simulink model "ROSsystem"  (R2021a)
settings: Solver=VariableStepAuto  StartTime=0.0  StopTime=10.0  RelTol=1e-3
values from neighbouring files (symbols this model uses):
  Fyf = zeros(1,57)    [FyfLookUpNewCar.m]    (also in Fyf_loopup_table.mat = [-9372.31873381 -9371.87234491 -9368.75632133 -9360.32413915)
  ks = 0    [controller_setup.m]
  SlipAngle = -SlipAngle    [FyfLookUpNewCar.m]    (also in Fyf_loopup_table.mat = [0.153111393254 0.147643129209 0.142174865164 0.13670660112 )
  Ts = 0.1    [controller_setup.m]
  Vx = 15    [controller_setup.m]
libraries: Solver_SF x1, simulink_extras x1, simulink x1
settings Model: Creator=chnwa  LastModifiedBy=chnwa

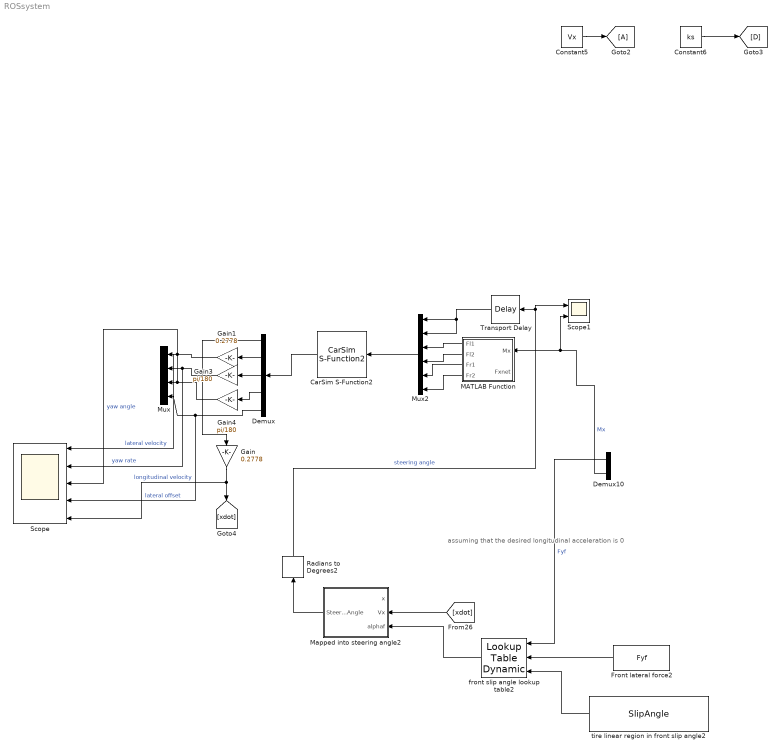
== system ROSsystem ==
  note: assuming that the desired longitudinal acceleration is 0
  CarSim S-Function2 : Solver_SF/CarSim S-Function2  Priority=1  VehicleCode=i_i  SIMFILE=simfile.sim
      settings: AttributesFormatString=Vehicle Code: %<VehicleCode>
  Constant5 : Constant  Value=Vx
  Constant6 : Constant  Value=ks
  Demux : Demux  Outputs=5
  Demux10 : Demux  Outputs=2
  Front lateral force2 : Constant  Value=Fyf
  Gain : Gain  Gain=0.2778
  Gain1 : Gain  Gain=0.2778
  Gain3 : Gain  Gain=pi/180
  Gain4 : Gain  Gain=pi/180
  MATLAB Function : MATLAB Function  TreatAsAtomicUnit=on
  Mapped into steering angle2 : MATLAB Function  TreatAsAtomicUnit=on
  Mux : Mux
  Mux2 : Mux  Inputs=6
  Radians to Degrees2 : simulink_extras/Transformations/Radians to Degrees
  Scope : Scope  NumInputPorts=5
  Scope1 : Scope  NumInputPorts=2
  Transport Delay : TransportDelay  DelayTime=Ts
  front slip angle lookup table2 : simulink/Lookup Tables/Lookup Table Dynamic  LookUpMeth=Interpolation-Use End Values  OutDataType=fixdt('double')  OutScaling=[]  OutputDataTypeScalingMode=Specify via dialog  OutDataTypeStr=double  DoSatur=off
  tire linear region in front slip angle2 : Constant  Value=SlipAngle
  wires:
  MATLAB Function/4(Fr2) -> Mux2/6
  Demux/1 -> Gain/1
  MATLAB Function/3(Fr1) -> Mux2/5
  Demux/2 -> Gain1/1
  MATLAB Function/2(Fl2) -> Mux2/4
  Gain4/1 -> Scope/3, Mux/3  "yaw angle"
  MATLAB Function/1(Fl1) -> Mux2/3
  Demux/3 -> Gain3/1
  Constant5/1 -> [A]
  Demux/5 -> Scope/4, Mux/4  "lateral offset"
  Mux2/1 -> CarSim S-Function2/1
  CarSim S-Function2/1 -> Demux/1
  Demux10/1 -> front slip angle lookup table2/1  "Fyf"
  Gain/1 -> [xdot], Scope/5  "longitudinal velocity"
  front slip angle lookup table2/1 -> Mapped into steering angle2/3(alphaf)
  Gain1/1 -> Scope/1, Mux/1  "lateral velocity"
  Constant6/1 -> [D]
  Demux/4 -> Gain4/1
  Gain3/1 -> Scope/2, Mux/2  "yaw rate"
  Front lateral force2/1 -> front slip angle lookup table2/2
  Transport Delay/1 -> Mux2/2, Mux2/1
  Radians to Degrees2/1 -> Transport Delay/1, Scope1/1  "steering angle"
  Mapped into steering angle2/1(SteeringAngle) -> Radians to Degrees2/1
  tire linear region in front slip angle2/1 -> front slip angle lookup table2/3
  Demux10/2 -> Scope1/2, MATLAB Function/1(Mx)  "Mx"
  [xdot] -> Mapped into steering angle2/2(Vx)

== matlab function ROSsystem/Mapped into steering angle2 ==
  data: x input; Vx input; alphaf input; SteeringAngle output
function SteeringAngle = fcn(x,Vx, alphaf)

lf = 1.11;  % distance from front axle to the mass center

Vy = x(1); %lateral velocity
r = x(2);  %yaw rate
SteeringAngle = Vy/Vx+lf*r/Vx-alphaf;

== matlab function ROSsystem/MATLAB Function ==
  data: Fl1 output; Mx input; Fl2 output; Fxnet input; Fr1 output; Fr2 output
function [Fl1,Fl2,Fr1,Fr2] = fcn(Mx,Fxnet)

w = 1.875; % the width of the car

Fwf = zeros(2,1);
Fwr = zeros(2,1);

if Mx > 0
    Fwf(1) = Fxnet/2+0;
    Fwf(2) = Fxnet/2-Mx/w;
    Fwr(1) = 0;
    Fwr(2) = -Mx/w;
elseif Mx < 0
    Fwf(1) = Fxnet/2+Mx/w;
    Fwf(2) = Fxnet/2+0;
    Fwr(1) = Mx/w;
    Fwr(2) = 0;
else
    Fwf(1) = Fxnet/2+0;
    Fwf(2) = Fxnet/2+0;
    Fwr(1) = 0;
    Fwr(2) = 0;
end
Fl1 = Fwf(1);
Fl2 = Fwr(1);
Fr1 = Fwf(2);
Fr2 = Fwr(2);
